simulink model "task4"  (R2016b)
settings: Solver=VariableStepAuto  StartTime=0.0  StopTime=30  RelTol=1e-3
undefined symbols (not defined in the file): eta_0, eta_d_0, eta_d_1, mu, s_0, U_ref
settings Model: Creator=Ørjan  LastModifiedBy=Ørjan

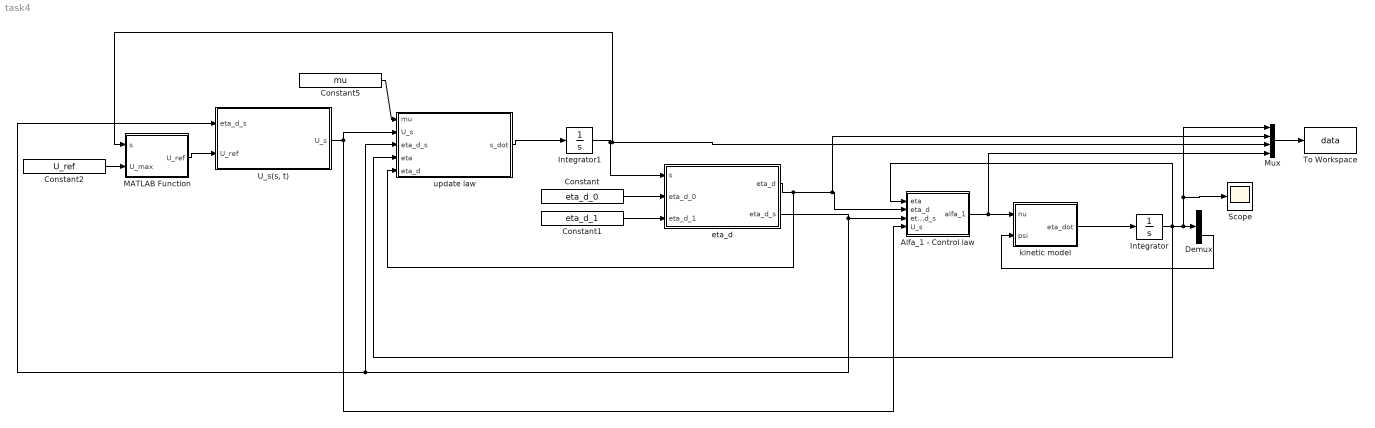
== system task4 ==
  Alfa_1 - Control law : MATLAB Function  TreatAsAtomicUnit=on
  Constant : Constant  Value=eta_d_0
  Constant1 : Constant  Value=eta_d_1
  Constant2 : Constant  Value=U_ref
  Constant5 : Constant  Value=mu
  Demux : Demux  Outputs=3
  Integrator : Integrator  InitialCondition=eta_0
  Integrator1 : Integrator  InitialCondition=s_0
  MATLAB Function : MATLAB Function  TreatAsAtomicUnit=on
  Mux : Mux
  Scope : Scope
  To Workspace : ToWorkspace  VariableName=data  SaveFormat=Timeseries  SampleTime=-1
      settings: Save2DSignal=2-D array (concatenate along first dimension)
  "U_s(s, t)" : MATLAB Function  TreatAsAtomicUnit=on
  eta_d : MATLAB Function  TreatAsAtomicUnit=on
  kinetic model : MATLAB Function  TreatAsAtomicUnit=on
  update law : MATLAB Function  TreatAsAtomicUnit=on
  wires:
  kinetic model/1(eta_dot) -> Integrator/1
  Integrator/1 -> update law/4(eta), Alfa_1 - Control law/1(eta), Scope/1, Mux/1, Demux/1
  Demux/3 -> kinetic model/2(psi)
  Alfa_1 - Control law/1(alfa_1) -> Mux/4, kinetic model/1(nu)
  update law/1(s_dot) -> Integrator1/1
  Integrator1/1 -> MATLAB Function/1(s), Mux/3, eta_d/1(s)
  eta_d/1(eta_d) -> update law/5(eta_d), Mux/2, Alfa_1 - Control law/2(eta_d)
  eta_d/2(eta_d_s) -> update law/3(eta_d_s), "U_s(s, t)"/1(eta_d_s), Alfa_1 - Control law/3(eta_d_s)
  Mux/1 -> To Workspace/1
  Constant/1 -> eta_d/2(eta_d_0)
  Constant1/1 -> eta_d/3(eta_d_1)
  "U_s(s, t)"/1(U_s) -> update law/2(U_s), Alfa_1 - Control law/4(U_s)
  Constant2/1 -> MATLAB Function/2(U_max)
  Constant5/1 -> update law/1(mu)
  MATLAB Function/1(U_ref) -> "U_s(s, t)"/2(U_ref)

== matlab function task4/Alfa_1 - Control law ==
  data: eta input; alfa_1 output; eta_d input; eta_d_s input; U_s input
function alfa_1 = fcn(eta, eta_d, eta_d_s, U_s)
K_p = diag([0.2 0.2 0.1]);

psi = eta(3);
R = [cos(psi) -sin(psi) 0; sin(psi) cos(psi) 0; 0 0 1];
z_1 = R'*(eta-eta_d);
alfa_1 = -K_p*z_1 + R'*eta_d_s*U_s;
end

== matlab function task4/kinetic model ==
  data: nu input; eta_dot output; psi input
function eta_dot  = R_psi(nu, psi)
eta_dot = [cos(psi) -sin(psi) 0; sin(psi) cos(psi) 0; 0 0 1]*nu;
end

== matlab function task4/U_s(s, t) ==
  data: U_s output size=1; eta_d_s input; U_ref input
function U_s = U_s(eta_d_s, U_ref)
U_s = abs(U_ref)/norm(eta_d_s(1:2), 2);
end

== matlab function task4/MATLAB Function ==
  data: s input; U_ref output; U_max input
function U_ref = fcn(s, U_max)
U_ref = U_max*(1.01 + sin(2*pi*s - pi/2));
end

== matlab function task4/eta_d ==
  data: eta_d output size=3; s input; eta_d_0 input; eta_d_1 input; eta_d_s output
function [eta_d, eta_d_s] = eta_d(s, eta_d_0, eta_d_1)
%% eta_d
x_d = (eta_d_1(1) - eta_d_0(1))*s + eta_d_0(1);
y_d = (eta_d_1(2) - eta_d_0(2))*s + eta_d_0(2);
psi_d = atan(y_d/x_d);
eta_d = [x_d; y_d; psi_d];

%% eta_d_s
x_d_s = eta_d_1(1) - eta_d_0(1);
y_d_s = eta_d_1(2) - eta_d_0(2);
psi_d_s = (y_d_s*eta_d(1) - eta_d(2)*x_d_s)/(eta_d(1)^2 + eta_d(2)^2);
eta_d_s = [x_d_s;y_d_s; psi_d_s];
end

== matlab function task4/update law ==
  data: mu input; s_dot output size=1; U_s input; eta_d_s input; eta input; eta_d input
function s_dot = s_dot(mu, U_s, eta_d_s, eta, eta_d)
psi = eta(3);

R_t = [cos(psi) -sin(psi) 0; sin(psi) cos(psi) 0; 0 0 1]';
z = R_t*(eta-eta_d);
V_1_s = -z'*R_t*eta_d_s;
s_dot = U_s - (mu/norm(eta_d_s, 2))*V_1_s;
end
